simulink subsystem "Phase1"  (R2023a)
settings: Solver=VariableStepAuto  StartTime=0.0  StopTime=10.0  RelTol=1e-3
values from neighbouring files (symbols this model uses):
  ikInitGuessSim = ikInitGuess    [defineTrajectory.m]
  P1_R1_waypoints = horzcat(initPosition,     [0.4000, 0, 0.8500 ... (first row only)    [defineTrajectory.m]
  P1_R1_waypointTimes = 0:3:6    [defineTrajectory.m]
  P1_R1_waypointVels = 0.1*[    1.5,  0,   1 ... (first row only)    [defineTrajectory.m]
libraries: robotcorelib x2, robotmaniplib x1
settings Model: Creator=lukasz  LastModifiedBy=lukasz

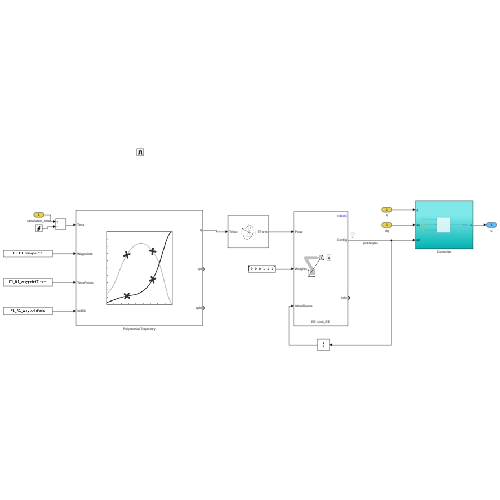
[thumbnail: Simulink's stored preview of the top-level diagram]
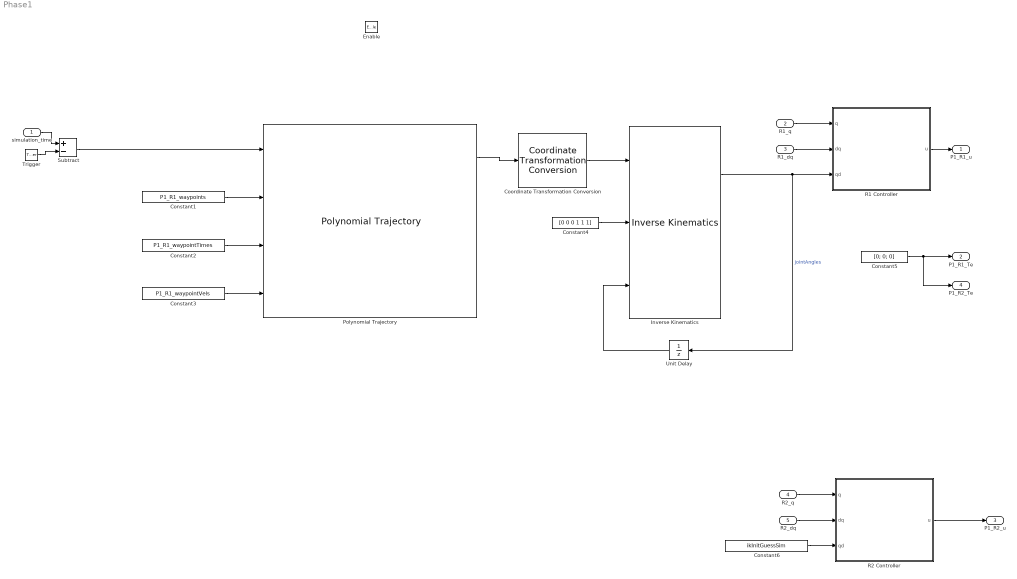
== system Phase1 ==
  simulation_time : Inport
  R1_q : Inport  Port=2
  R1_dq : Inport  Port=3
  R2_q : Inport  Port=4
  R2_dq : Inport  Port=5
  Enable : EnablePort
  Trigger : TriggerPort  VariantControl=(inherit)  ShowOutputPort=on
  Constant1 : Constant  Value=P1_R1_waypoints  VectorParams1D=off  SampleTime=-1
  Constant2 : Constant  Value=P1_R1_waypointTimes  VectorParams1D=off  SampleTime=-1
  Constant3 : Constant  Value=P1_R1_waypointVels  VectorParams1D=off  SampleTime=-1
  Constant4 : Constant  Value=[0 0 0 1 1 1]  VectorParams1D=off
  Constant5 : Constant  Value=[0; 0; 0]  VectorParams1D=off
  Constant6 : Constant  Value=ikInitGuessSim  VectorParams1D=off  SampleTime=-1
  Coordinate Transformation Conversion : robotcorelib/Coordinate Transformation Conversion  InputRepresentation=Translation Vector  InputEulerSequence=ZYX  ShowTrVecInputPort=on  OutputRepresentation=Homogeneous Transformation  OutputEulerSequence=ZYX  ShowTrVecOutputPort=on  SimulateUsing=Code generation
  Inverse Kinematics : robotmaniplib/Inverse Kinematics  RigidBodyTree=robot1  EndEffector=Link_EE  ShowInfo=on  SolverName=BFGS Gradient Projection  EnforceJointLimits=on  MaxIterations=1500  MaxTime=10  GradientTolerance=1e-7  SolutionTolerance=1e-6  StepTolerance=1e-14  ErrorChangeTolerance=1e-12  UseErrorDamping=on  DampingBias=0.0025  SimulateUsing=Code generation
  Polynomial Trajectory : robotcorelib/Polynomial Trajectory  WaypointSource=External  Waypoints=[ 0, 2, 1, 5, 0; -1, 3, 1, 4, 4 ]  TimePoints=[ 0, 1, 2, 3, 4 ]  TimeInterval=[ 1, 4 ]  Method=Cubic Polynomial  ParameterSource=External  VelocityBoundaryCondition=zeros( 2, 5 )  AccelerationBoundaryCondition=zeros( 2, 5 )  SimulateUsing=Interpreted execution
  R1 Controller : Subsystem
  R2 Controller : Subsystem
  Subtract : Sum  Inputs=+-
  Unit Delay : UnitDelay  InitialCondition=ikInitGuessSim  SampleTime=-1  HasFrameUpgradeWarning=on
  P1_R1_u : Outport
  P1_R1_Te : Outport  Port=2
  P1_R2_u : Outport  Port=3
  P1_R2_Te : Outport  Port=4
  wires:
  Subtract/1 -> Polynomial Trajectory/1
  simulation_time/1 -> Subtract/1
  Trigger/1 -> Subtract/2
  Constant1/1 -> Polynomial Trajectory/2
  Constant2/1 -> Polynomial Trajectory/3
  Constant3/1 -> Polynomial Trajectory/4
  Polynomial Trajectory/1 -> Coordinate Transformation Conversion/1
  Unit Delay/1 -> Inverse Kinematics/3
  Constant4/1 -> Inverse Kinematics/2
  Coordinate Transformation Conversion/1 -> Inverse Kinematics/1
  Inverse Kinematics/1 -> R1 Controller/3(qd), Unit Delay/1  "jointAngles"
  R1_q/1 -> R1 Controller/1(q)
  R1_dq/1 -> R1 Controller/2(dq)
  R1 Controller/1(u) -> P1_R1_u/1
  Constant5/1 -> P1_R1_Te/1, P1_R2_Te/1
  R2_q/1 -> R2 Controller/1(q)
  R2_dq/1 -> R2 Controller/2(dq)
  R2 Controller/1(u) -> P1_R2_u/1
  Constant6/1 -> R2 Controller/3(qd)

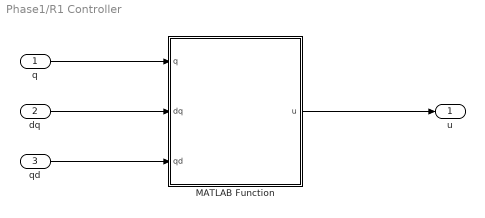
== system Phase1/R1 Controller ==
  q : Inport
  dq : Inport  Port=2
  qd : Inport  Port=3
  MATLAB Function : MATLAB Function  TreatAsAtomicUnit=on
  u : Outport
  wires:
  dq/1 -> MATLAB Function/2(dq)
  MATLAB Function/1(u) -> u/1
  qd/1 -> MATLAB Function/3(qd)
  q/1 -> MATLAB Function/1(q)

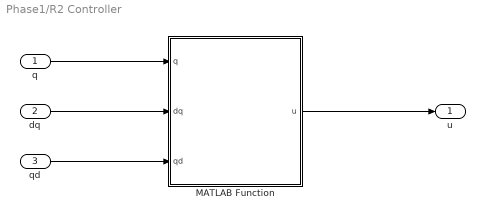
== system Phase1/R2 Controller ==
  q : Inport
  dq : Inport  Port=2
  qd : Inport  Port=3
  MATLAB Function : MATLAB Function  TreatAsAtomicUnit=on
  u : Outport
  wires:
  dq/1 -> MATLAB Function/2(dq)
  MATLAB Function/1(u) -> u/1
  qd/1 -> MATLAB Function/3(qd)
  q/1 -> MATLAB Function/1(q)

== matlab function Phase1/R2 Controller/MATLAB Function ==
  data: q input; dq input; u output; qd input
function u = fcn(q, dq, qd)
% PD + gravity compensation controller function

%% general physical parameters

l1 = 0.6731;
l2 = 0.432;
l3 = 0.434;
lc2 = 0.216;
lc3 = 0.164;
m2 = 15.46;
m3 = 9.55;
J = 0.302;

%% Joint Space variables

q1 = q(1);
q2 = q(2);
q3 = q(3);

dq1 = dq(1);
dq2 = dq(2);
dq3 = dq(3);
g = 9.81;

%% Vector of Potential Forces Parameters

g21 = -g * (lc3 * m3 * sin(q2 + q3) + lc2 * m2 * cos(q2) + l2 * m3 * cos(q2));
g31 = -g * (lc3 * m3 * sin(q2 + q3));

G = [0;
    g21;
    g31];

%% PD Controller Parameters 

Kp = [20,0,0; 0, 10 ,0; 0, 0 , 10];  %  Kp is 3*3 matrix of proportional gain 
Kd = [1,0,0; 0, 1 ,0; 0, 0 , 1]; %Kd is 3*3 matrix of derivative gain

%% Control law

u = - Kp * (q - qd) - Kd * dq + G;

== matlab function Phase1/R1 Controller/MATLAB Function ==
  data: q input; dq input; u output; qd input
function u = fcn(q, dq, qd)
% PD + gravity compensation controller function

%% general physical parameters

l1 = 0.6731;
l2 = 0.432;
l3 = 0.434;
lc2 = 0.216;
lc3 = 0.164;
m2 = 15.46;
m3 = 9.55;
J = 0.302;

%% Joint Space variables

q1 = q(1);
q2 = q(2);
q3 = q(3);

dq1 = dq(1);
dq2 = dq(2);
dq3 = dq(3);
g = 9.81;

%% Vector of Potential Forces Parameters

g21 = -g * (lc3 * m3 * sin(q2 + q3) + lc2 * m2 * cos(q2) + l2 * m3 * cos(q2));
g31 = -g * (lc3 * m3 * sin(q2 + q3));

G = [0;
    g21;
    g31];

%% PD Controller Parameters 

Kp = [10,0,0; 0, 10 ,0; 0, 0 , 10];  %  Kp is 3*3 matrix of proportional gain 
Kd = [1,0,0; 0, 1 ,0; 0, 0 , 1]; %Kd is 3*3 matrix of derivative gain

%% Control law

u = - Kp * (q - qd) - Kd * dq + G;
